simulink library "EmptyTranslationEngine"  (R2022b)
settings: Solver=VariableStepAuto  StartTime=0.0  StopTime=10.0  RelTol=1e-3
undefined symbols (not defined in the file or in its folder): Row
libraries: TuneVar x2, FeaturePath x1, TOP x1
settings Model: MAModelExclusionFileProxy=C:\work\talariaDev\module\talaria_check_exclusions.xml  Creator=kl13806  LastModifiedBy=kl13806
settings SolverCC: AlgebraicLoopSolver=TrustRegion
settings DebuggingCC: UnconnectedInputMsg=warning  UnconnectedOutputMsg=warning  UnconnectedLineMsg=warning  SFMachineParentedDataDiag=warning  ArithmeticOperatorsInVariantConditions=warning
settings ModelReferenceCC: EnableRefExpFcnMdlSchedulingChecks=on
settings SFSimCC: SimUseLocalCustomCode=off  CustomCodeUndefinedFunction=UseInterfaceOnly
settings RTWCC: RTWUseLocalCustomCode=off  DLArmComputeVersion=19.05

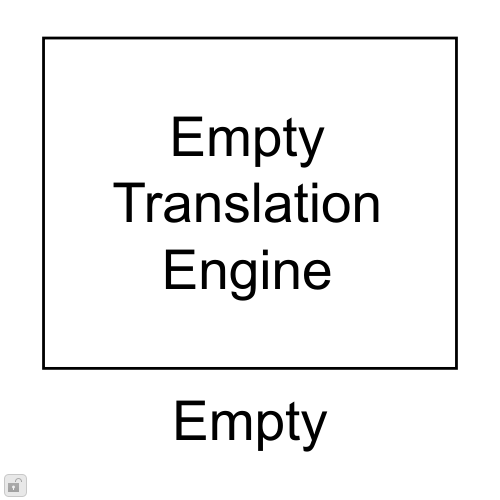
[thumbnail: Simulink's stored preview of the top-level diagram]
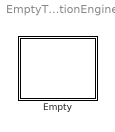
== system EmptyTranslationEngine ==
  Empty : Subsystem  mask(Talaria Empty Translation Engine){}
      mask Display: disp(['Empty' newline 'Translation' newline 'Engine']);

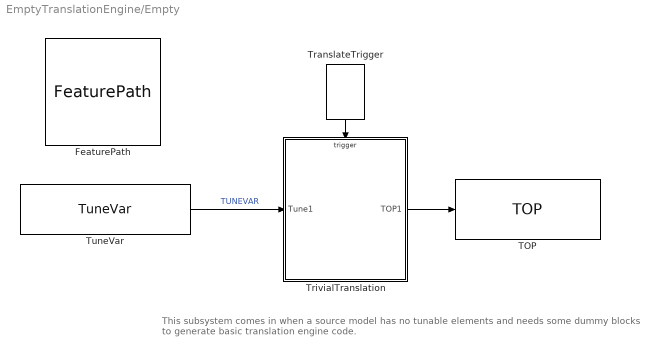
== system EmptyTranslationEngine/Empty ==
  note: This subsystem comes in when a source model
      | has no tunable elements and needs some dummy
      | blocks to generate basic translation engine code.
  FeaturePath : FeaturePath/FeaturePath  FeatureName=DUMMY_  IsGroup=on  GroupNumber=-1  IsModule=off  TriggerInit=[45 19 160 126]
      settings: SourceProductName=Bose Talaria
  TOP : TOP/TOP  TriggerInit=[455 160 600 220]  TopName=TOP  DataType=single  BankNumber=0  PreOverlay=false  PostOverlay=false  Role=Automatic
      settings: SourceProductName=Bose Talaria
  TranslateTrigger : TuneVar/TranslateTrigger  TriggerInit=[241 80 279 135]
      settings: SourceProductName=Bose Talaria
  TrivialTranslation : MATLAB Function  TreatAsAtomicUnit=on  mask(Talaria Trivial Translation){}
  TuneVar : TuneVar/TuneVar  TuneName=TUNEVAR  SpecifyMaxSize=off  VariableDim=1 (Row)  MaxSize=[1 1]  TunabilityNumber=1  MinValue=[]  MaxValue=[]  TriggerInit=[20 165 190 215]  MaskValue=[1]
      settings: SourceProductName=Bose Talaria
  wires:
  TranslateTrigger/1 -> TrivialTranslation/Trigger
  TrivialTranslation/1(TOP1) -> TOP/1
  TuneVar/1 -> TrivialTranslation/1(Tune1)  "TUNEVAR"

== matlab function EmptyTranslationEngine/Empty/TrivialTranslation ==
  data: TOP1 output; Tune1 input
  events: trigger input FUNCTION_CALL_EVENT
function TOP1  = fcn(Tune1)
%#codegen

% ----- To access TuneVar maximum size, current size, and current value:
%   Note: TuneVar signals arrive with exposed variable size information.
%         The expressions below illustrate for the "Tune1" input argument.
%
%   size(Tune1.Value) : the maximum possible size of the Tune1 variable
%
%   Tune.Size   : the current size of *valid* data in Tune1.Value
%
%   Tune1.Size(1) : Number of rows present in Tune1 - this does not vary.
%
%   Tune1.Size(2) : Number of columns currently valid in Tune1 - this is
%       the variable part of size that can change (if allowed by TuneVar).
%
%   Tune1.Value : the current value of the tune variable... but end-padded 
%       to the maximum available size with undefined/invalid data.
%
%   numel(Tune1.Value) : another way of looking at the maximum number of
%       elements that could arrive in Tune1.Value
%
% ----- To register an error, use the following method (works like printf):
%   TranslateError( <format string>, <arguments ... )
%   ... this error will cause the build process to abort.

% A trivial pass-through translation looks like this:
TOP1 = Tune1.Value;
